simulink model "pendule"  (R2022b)
settings: Solver=VariableStepAuto  StartTime=0.0  StopTime=10.0  RelTol=1e-3
undefined symbols (not defined in the file): G, l
settings Model: Creator=mathissigier  LastModifiedBy=mathissigier

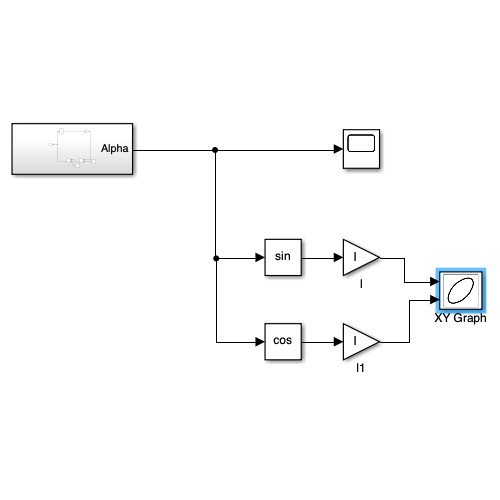
[thumbnail: Simulink's stored preview of the top-level diagram]
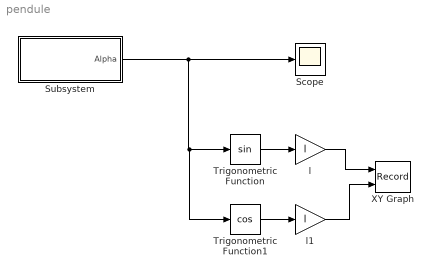
== system pendule ==
  Scope : Scope
  Subsystem : Subsystem
  Trigonometric Function : Trigonometry
  Trigonometric Function1 : Trigonometry  Operator=cos
  XY Graph : Record  FileSettingsInternal="{\"entries\":[{\"content\":{\"excelSettings\":{\"content\":{},\"type\":\"Streamout.ExcelSettings\"}},\"type\":\"Streamout.FileSettingStorage\",\"uuid\":\"bfaeb260-ec50-400a-81fc-0bdf14d035d5\"}],\"packageUris\":[\"http://schema.mathworks.com/mf0/streamout_blocks/R2020a\"],\"version\":\"1.0\"}"  Layout=[1 1]  SignalsInternal="{\"entries\":[{\"content\":{\"signals\":[{\"content\":{\"blockPath\":[\"pendule/XY Graph\"],\"channel\":[],\"dimensions\":[1],\"domain\":\"pendule/XY Graph\",\"lineColor\":\"#a2142f\",\"plots\":[1],\"port\":1,\"sid\":[\"\"],\"signalID\":210,\"signalName\":\"l\"},\"type\":\"RecordBlkView.Signal\",\"uuid\":\"ef09d82d-3276-4fd6-a865-e9a13a28aad2\"},{\"content\":{\"blockPath\":[\"pendule/XY Graph\"],\"channel\":[],\"dimensions\":[1],\"domain\":\"pendule/XY Graph\",\"lineColor\":\"#139fff\",\"plots\":[1],\"port\":2,\"sid\":[\"\"],\"signalID\":214,\"signalName\":\"l1\"},\"type\":\"RecordBlkView.Signal\",\"uuid\":\"c71a7022-60e1-4877-ba63-4b2b9dd38011\"}]},\"type\":\"RecordBlkView.InputSignals\",\"uuid\":\"3120cf51-4e08-485d-abdf-24d7701eb1d7\"}],\"packageUris\":[\"http://schema.mathworks.com/mf0/streamout_blocks/R2020a\"],\"version\":\"1.0\"}"  VisualizationBindings="{\"xyplotplugin\":{\"info\":[{\"series\":[{\"bindingParametersList\":[{\"parameter\":\"X-Axis\",\"signalID\":210,\"signalName\":\"l\"},{\"parameter\":\"Y-Axis\",\"signalID\":214,\"signalName\":\"l1\"}],\"seriesID\":62685}],\"subplotID\":1}]}}"  CompatibilityTag=XY
  l : Gain  Gain=l
  l1 : Gain  Gain=l
  wires:
  Subsystem/1(Alpha) -> Trigonometric Function1/1, Trigonometric Function/1, Scope/1
  Trigonometric Function/1 -> l/1
  Trigonometric Function1/1 -> l1/1
  l/1 -> XY Graph/1
  l1/1 -> XY Graph/2

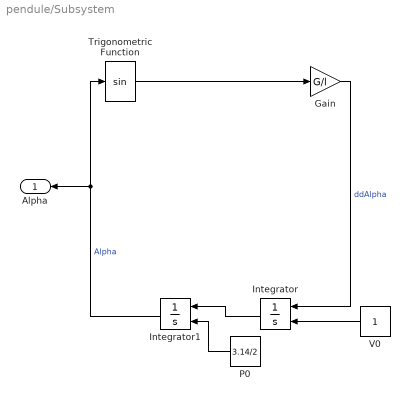
== system pendule/Subsystem ==
  Gain : Gain  Gain=G/l
  Integrator : Integrator  InitialConditionSource=external
  Integrator1 : Integrator  InitialConditionSource=external
  P0 : Constant  Value=3.14/2
  Trigonometric Function : Trigonometry
  V0 : Constant
  Alpha : Outport
  wires:
  Integrator1/1 -> Alpha/1, Trigonometric Function/1  "Alpha"
  Integrator/1 -> Integrator1/1
  V0/1 -> Integrator/2
  P0/1 -> Integrator1/2
  Trigonometric Function/1 -> Gain/1
  Gain/1 -> Integrator/1  "ddAlpha"
